simulink model "DIPCalt"  (R2015a)
settings: Solver=ode3  SolverMode=SingleTasking  StartTime=0.0  StopTime=5  FixedStep=1e-3  RelTol=1e-3
values from neighbouring files (symbols this model uses):
  deltas = ds/20    (= 45)    [DIPCinit.m]
  deltav = 1500    [DIPCinit.m]
  ds = 900    [DIPCinit.m]
  dv = 1500    [DIPCinit.m]
  g = [0;0;0]    [DIPCinit.m]
  j0 = 0.2    [DIPCinit.m]
  j1 = 0.5    [DIPCinit.m]
  j2 = 0.5    [DIPCinit.m]
  j3 = 0.5    [DIPCinit.m]
  j4 = 0.5    [DIPCinit.m]
  jiv = 0.5    [DIPCinit.m]
  jv = j0*1    (= 0.2)    [DIPCinit.m]
  kappas = ks/20    (= 9)    [DIPCinit.m]
  kappav = 700    [DIPCinit.m]
  ks = 180    [DIPCinit.m]
  kv = 700    [DIPCinit.m]
  m0 = 1.4    [DIPCinit.m]
  m1 = 10    [DIPCinit.m]
  m2 = 10    [DIPCinit.m]
  m3 = 10    [DIPCinit.m]
  m4 = 10    [DIPCinit.m]
  miv = 10    [DIPCinit.m]
  mv = m0*1    (= 1.4)    [DIPCinit.m]
  r = 0.4*[1 0 0 0 1 0 -1 0 0 0 -1 0]'    [DIPCinit.m]
libraries: aerolibutil x20, dspinverses x4, simulink x3, aerolibtransform2 x2
(part 1 of 2)
settings Model: CovSFcnEnable=off  Creator=Martin  LastModifiedBy=mangerer
settings OptimizationCC: BlockReduction=off  BooleanDataType=off  OptimizeBlockIOStorage=off  BufferReuse=off  GlobalBufferReuse=off  ExpressionFolding=off  LocalBlockOutputs=off
settings DebuggingCC: SaveWithParameterizedLinksMsg=none  UnderspecifiedInitializationDetection=Classic  MergeDetectMultiDrivingBlocksExec=none  SignalResolutionControl=TryResolveAllWithWarning
settings HardwareCC: TargetUnknown=on

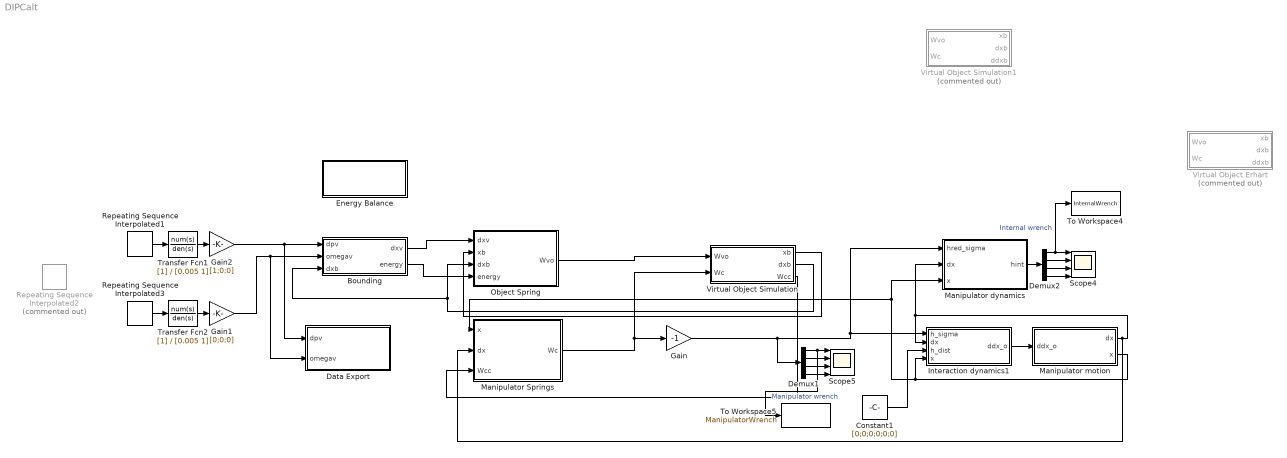
== system DIPCalt ==
  Bounding : Subsystem
  Constant1 : Constant  Value=[0;0;0;0;0;0]
  Data Export : Subsystem
  Demux1 : Demux
  Demux2 : Demux
  Energy Balance : Subsystem
  Gain : Gain  Gain=-1
  Gain1 : Gain  Gain=[0;0;0]
  Gain2 : Gain  Gain=[1;0;0]
  Interaction dynamics1 : Subsystem
  Manipulator Springs : Subsystem
  Manipulator dynamics : Subsystem
  Manipulator motion : Subsystem
  Object Spring : Subsystem
  Repeating Sequence Interpolated1 : simulink/Sources/Repeating Sequence Interpolated  OutValues="[0 0 0.2 0, 0 1 0, 0  -0.5 0, 0].'"  TimeValues=5/3*[0 0.1 0.25 0.4, 0.5 1.2 1.95, 2.15 2.45 2.85, 3].'  LookUpMeth=Interpolation-Use End Values  tsamp=0.001  OutMin=[]  OutMax=[]  OutDataTypeStr=double  OutputDataTypeScalingMode=double  OutDataType=fixdt(0,8)  OutScaling=2^-10
  Repeating Sequence Interpolated2 : simulink/Sources/Repeating Sequence Interpolated  Commented=on  OutValues=[0 0 2 2 -0.5 -0.5 0 0].'  TimeValues=[0 0.1 1 1.3 1.9 2.2 2.7 3].'  LookUpMeth=Interpolation-Use End Values  tsamp=0.001  OutMin=[]  OutMax=[]  OutDataTypeStr=double  OutputDataTypeScalingMode=double  OutDataType=fixdt(0,8)  OutScaling=2^-10
  Repeating Sequence Interpolated3 : simulink/Sources/Repeating Sequence Interpolated  OutValues="[0 0 0.2 0, 0 1 0, 0  -0.5 0, 0].'"  TimeValues=5/3*[0 0.1 0.25 0.4, 0.5 1.2 1.95, 2.15 2.45 2.85, 3].'  LookUpMeth=Interpolation-Use End Values  tsamp=0.001  OutMin=[]  OutMax=[]  OutDataTypeStr=double  OutputDataTypeScalingMode=double  OutDataType=fixdt(0,8)  OutScaling=2^-10
  Scope4 : Scope  NumInputPorts=4
      settings: ShowLegends=on  TimeRange=5  YMin=-2.25~-2.25~-1.5~-1.5  YMax=1.5~1.5~2.25~2.25  SaveName=ScopeData6
  Scope5 : Scope  NumInputPorts=4
      settings: ShowLegends=on  TimeRange=5  YMin=-12.5~-12.5~-20~-20  YMax=20~20~12.5~12.5  SaveName=ScopeData11
  To Workspace4 : ToWorkspace  VariableName=InternalWrench  SaveFormat=Timeseries  SampleTime=-1
  To Workspace5 : ToWorkspace  VariableName=ManipulatorWrench  SaveFormat=Timeseries  SampleTime=-1
  Transfer Fcn1 : TransferFcn  Denominator=[0.005 1]
  Transfer Fcn2 : TransferFcn  Denominator=[0.005 1]
  Virtual Object Erhart : Subsystem  Commented=on
  Virtual Object Simulation : Subsystem
  Virtual Object Simulation1 : Subsystem  Commented=on
  wires:
  Object Spring/1(Wvo) -> Virtual Object Simulation/1(Wvo)
  Virtual Object Simulation/1(xb) -> Object Spring/2(xb)
  Manipulator Springs/1(Wc) -> Virtual Object Simulation/2(Wc), Gain/1
  Interaction dynamics1/1(ddx_o) -> Manipulator motion/1(ddx_o)
  Constant1/1 -> Interaction dynamics1/3(h_dist)
  Manipulator motion/1(dx) -> Manipulator Springs/2(dx), Manipulator dynamics/2(dx), Interaction dynamics1/2(dx)
  Manipulator motion/2(x) -> Manipulator dynamics/3(x), Manipulator Springs/1(x), Interaction dynamics1/4(x)
  Virtual Object Simulation/2(dxb) -> Object Spring/3(dxb), Bounding/3(dxb)
  Manipulator dynamics/1(hint) -> Demux2/1
  Demux2/2 -> Scope4/2
  Demux2/4 -> Scope4/4
  Demux2/3 -> Scope4/3
  Demux2/1 -> To Workspace4/1, Scope4/1  "Internal wrench"
  Repeating Sequence Interpolated1/1 -> Transfer Fcn1/1
  Transfer Fcn1/1 -> Gain2/1
  Transfer Fcn2/1 -> Gain1/1
  Gain/1 -> Demux1/1, Manipulator dynamics/1(hred_sigma), Interaction dynamics1/1(h_sigma)
  Demux1/2 -> Scope5/2
  Demux1/4 -> Scope5/4
  Demux1/3 -> Scope5/3
  Demux1/1 -> To Workspace5/1, Scope5/1  "Manipulator wrench"
  Gain1/1 -> Data Export/2(omegav), Bounding/2(omegav)
  Gain2/1 -> Data Export/1(dpv), Bounding/1(dpv)
  Bounding/1(dxv) -> Object Spring/1(dxv)
  Bounding/2(energy) -> Object Spring/4(energy)
  Repeating Sequence Interpolated3/1 -> Transfer Fcn2/1
  Virtual Object Simulation/3(Wcc) -> Manipulator Springs/3(Wcc)

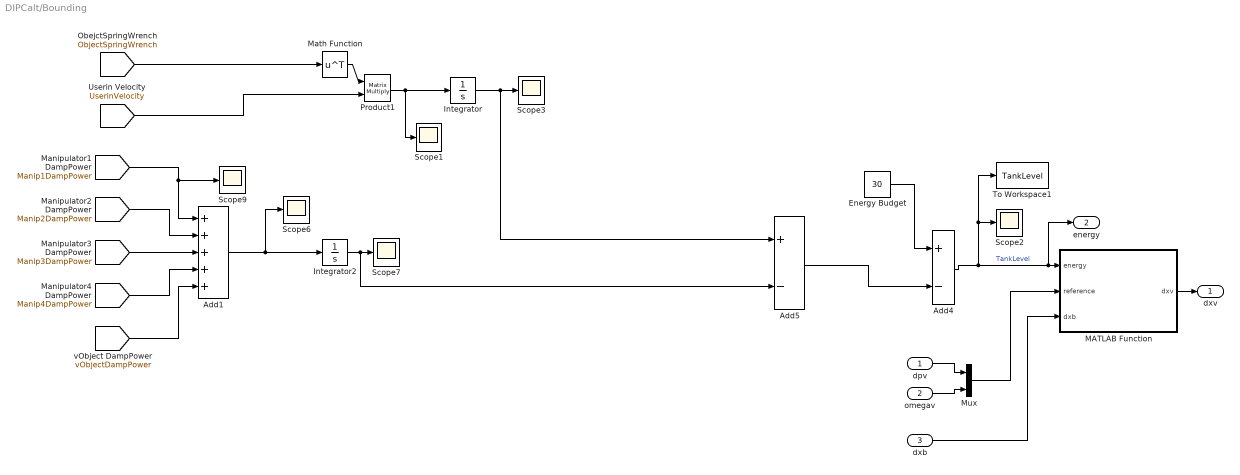
== system DIPCalt/Bounding ==
  dpv : Inport
  omegav : Inport  Port=2
  dxb : Inport  Port=3
  Add1 : Sum  Inputs=+++++
  Add4 : Sum  Inputs=+-
  Add5 : Sum  Inputs=+-
  Energy Budget : Constant  Value=30
  Integrator : Integrator
  Integrator2 : Integrator
  MATLAB Function : MATLAB Function  TreatAsAtomicUnit=on
  Math Function : Math  Operator=transpose  SaturateOnIntegerOverflow=on
  Mux : Mux  Inputs=2
  Product1 : Product  Multiplication=Matrix(*)
  Scope{1..3,6..7,9} (6 alike) : Scope
      Scope1 settings: YMin=0  YMax=60  SaveName=ScopeData5
      Scope2 settings: TimeRange=4.999  YMin=19.5  YMax=30
      Scope3 settings: YMin=0  YMax=15  SaveName=ScopeData14
      Scope6 settings: YMin=-0.3  YMax=0.05  SaveName=ScopeData40
      Scope7 settings: YMin=675  YMax=1000  SaveName=ScopeData41
      Scope9 settings: YMin=0  YMax=3e-05  SaveName=ScopeData46
  To Workspace1 : ToWorkspace  VariableName=TankLevel  SaveFormat=Timeseries  SampleTime=-1
  dxv : Outport
  energy : Outport  Port=2
  wires:
  Energy Budget/1 -> Add4/1
  Add4/1 -> energy/1, MATLAB Function/1(energy), To Workspace1/1, Scope2/1  "TankLevel"
  dpv/1 -> Mux/1
  omegav/1 -> Mux/2
  Mux/1 -> MATLAB Function/2(reference)
  dxb/1 -> MATLAB Function/3(dxb)
  MATLAB Function/1(dxv) -> dxv/1
  Product1/1 -> Integrator/1, Scope1/1
  [UserinVelocity] -> Product1/2
  Integrator/1 -> Add5/1, Scope3/1
  [Manip1DampPower] -> Scope9/1, Add1/1
  [Manip2DampPower] -> Add1/2
  [Manip3DampPower] -> Add1/3
  [Manip4DampPower] -> Add1/4
  [vObjectDampPower] -> Add1/5
  Add1/1 -> Integrator2/1, Scope6/1
  Integrator2/1 -> Add5/2, Scope7/1
  Math Function/1 -> Product1/1
  [ObjectSpringWrench] -> Math Function/1
  Add5/1 -> Add4/2

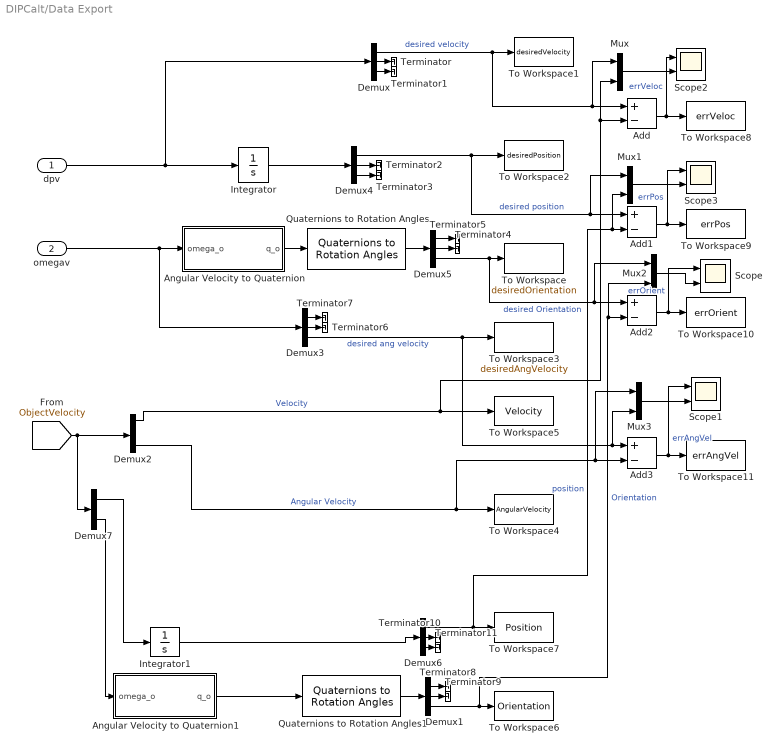
== system DIPCalt/Data Export ==
  dpv : Inport
  omegav : Inport  Port=2
  Add{,1..3} (4 alike) : Sum  Inputs=+-
  Angular Velocity to Quaternion : Subsystem
  Angular Velocity to Quaternion1 : Subsystem
  Demux{,1,3..6} (6 alike) : Demux  Outputs=3
  Demux2 : Demux  Outputs=6
  Demux7 : Demux  Outputs=2
  Integrator : Integrator
  Integrator1 : Integrator  InitialCondition=[0 0 0]'
  Mux{,1..3} (4 alike) : Mux  Inputs=2
  Quaternions to Rotation Angles : aerolibtransform2/Quaternions to Rotation Angles  rotationOrder=XYZ
  Quaternions to Rotation Angles1 : aerolibtransform2/Quaternions to Rotation Angles  rotationOrder=XYZ
  Scope{,1..3} (4 alike) : Scope  NumInputPorts=2
      Scope settings: YMin=-0.0005~-5  YMax=0.0025~5  SaveName=ScopeData13
      Scope1 settings: YMin=-0.06~-0.025  YMax=0.08~0.225  SaveName=ScopeData37
      Scope2 settings: TimeRange=4.999  YMin=-0.3~-0.5  YMax=0.2~1  SaveName=ScopeData19
      Scope3 settings: YMin=-0.0005~-5  YMax=0.0025~5  SaveName=ScopeData39
  Terminator{,1..11} (12 alike) : Terminator
  To Workspace : ToWorkspace  VariableName=desiredOrientation  SaveFormat=Timeseries  SampleTime=-1
  To Workspace1 : ToWorkspace  VariableName=desiredVelocity  SaveFormat=Timeseries  SampleTime=-1
  To Workspace10 : ToWorkspace  VariableName=errOrient  SaveFormat=Timeseries  SampleTime=-1
  To Workspace11 : ToWorkspace  VariableName=errAngVel  SaveFormat=Timeseries  SampleTime=-1
  To Workspace2 : ToWorkspace  VariableName=desiredPosition  SaveFormat=Timeseries  SampleTime=-1
  To Workspace3 : ToWorkspace  VariableName=desiredAngVelocity  SaveFormat=Timeseries  SampleTime=-1
  To Workspace4 : ToWorkspace  VariableName=AngularVelocity  SaveFormat=Timeseries  SampleTime=-1
  To Workspace5 : ToWorkspace  VariableName=Velocity  SaveFormat=Timeseries  SampleTime=-1
  To Workspace6 : ToWorkspace  VariableName=Orientation  SaveFormat=Timeseries  SampleTime=-1
  To Workspace7 : ToWorkspace  VariableName=Position  SaveFormat=Timeseries  SampleTime=-1
  To Workspace8 : ToWorkspace  VariableName=errVeloc  SaveFormat=Timeseries  SampleTime=-1
  To Workspace9 : ToWorkspace  VariableName=errPos  SaveFormat=Timeseries  SampleTime=-1
  wires:
  Demux4/1 -> Mux1/1, Add1/1, To Workspace2/1  "desired position"
  Demux/1 -> Mux/1, Add/1, To Workspace1/1  "desired velocity"
  Integrator/1 -> Demux4/1
  dpv/1 -> Demux/1, Integrator/1
  Demux/2 -> Terminator/1
  Demux/3 -> Terminator1/1
  Demux4/2 -> Terminator2/1
  Demux4/3 -> Terminator3/1
  Quaternions to Rotation Angles/1 -> Demux5/1
  Demux5/3 -> Mux2/1, Add2/1, To Workspace/1  "desired Orientation"
  Demux3/3 -> Mux3/2, Add3/1, To Workspace3/1  "desired ang velocity"
  Angular Velocity to Quaternion/1(q_o) -> Quaternions to Rotation Angles/1
  omegav/1 -> Demux3/1, Angular Velocity to Quaternion/1(omega_o)
  Demux5/2 -> Terminator4/1
  Demux5/1 -> Terminator5/1
  Demux3/2 -> Terminator6/1
  Demux3/1 -> Terminator7/1
  Demux2/1 -> Mux/2, Add/2, To Workspace5/1  "Velocity"
  Demux2/6 -> Mux3/1, Add3/2, To Workspace4/1  "Angular Velocity"
  [ObjectVelocity] -> Demux7/1, Demux2/1
  Quaternions to Rotation Angles1/1 -> Demux1/1
  Demux1/3 -> Mux2/2, Add2/2, To Workspace6/1  "Orientation"
  Demux1/2 -> Terminator9/1
  Demux1/1 -> Terminator8/1
  Demux6/1 -> Mux1/2, Add1/2, To Workspace7/1  "position"
  Demux6/2 -> Terminator10/1
  Demux6/3 -> Terminator11/1
  Demux7/1 -> Integrator1/1
  Integrator1/1 -> Demux6/1
  Demux7/2 -> Angular Velocity to Quaternion1/1(omega_o)
  Angular Velocity to Quaternion1/1(q_o) -> Quaternions to Rotation Angles1/1
  Add/1 -> Scope2/1, To Workspace8/1  "errVeloc"
  Add1/1 -> Scope3/1, To Workspace9/1  "errPos"
  Add2/1 -> Scope/1, To Workspace10/1  "errOrient"
  Add3/1 -> Scope1/1, To Workspace11/1  "errAngVel"
  Mux/1 -> Scope2/2
  Mux1/1 -> Scope3/2
  Mux2/1 -> Scope/2
  Mux3/1 -> Scope1/2

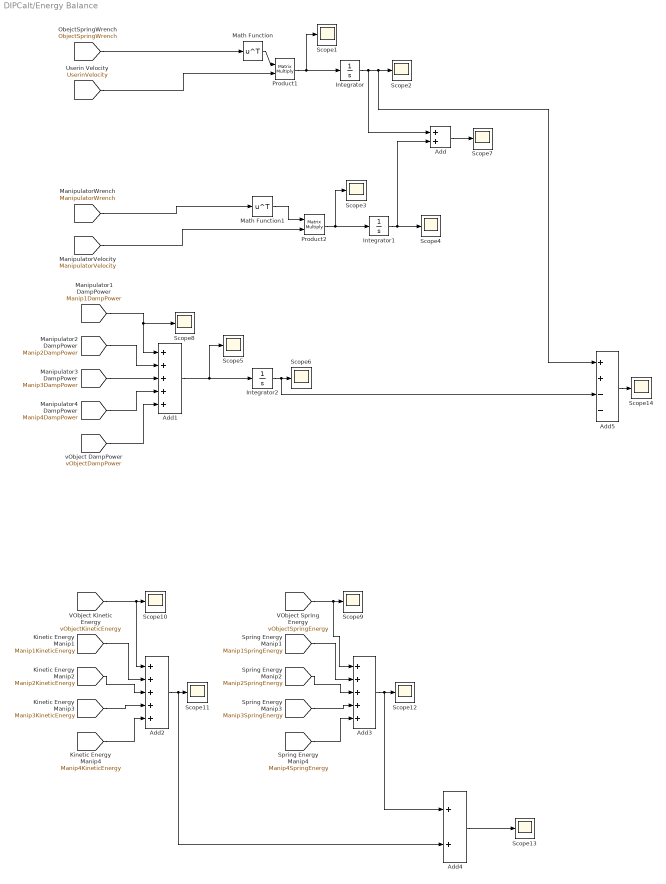
== system DIPCalt/Energy Balance ==
  Add : Sum
  Add1 : Sum  Inputs=+++++
  Add2 : Sum  Inputs=+++++
  Add3 : Sum  Inputs=+++++
  Add4 : Sum
  Add5 : Sum  Inputs=++--
  Integrator : Integrator
  Integrator1 : Integrator
  Integrator2 : Integrator
  Math Function : Math  Operator=transpose  SaturateOnIntegerOverflow=on
  Math Function1 : Math  Operator=transpose  SaturateOnIntegerOverflow=on
  Product1 : Product  Multiplication=Matrix(*)
  Product2 : Product  Multiplication=Matrix(*)
  Scope{1..14} (14 alike) : Scope
      Scope1 settings: YMin=0  YMax=60  SaveName=ScopeData24
      Scope10 settings: YMin=0  YMax=0.08  SaveName=ScopeData29
      Scope11 settings: YMin=0  YMax=12  SaveName=ScopeData30
      Scope12 settings: YMin=0  YMax=0.00021  SaveName=ScopeData31
      Scope13 settings: YMin=0  YMax=50  SaveName=ScopeData32
      Scope14 settings: YMin=0  YMax=42.5  SaveName=ScopeData33
      Scope2 settings: YMin=0  YMax=15  SaveName=ScopeData18
      Scope3 settings: YMin=-60  YMax=10  SaveName=ScopeData20
      Scope4 settings: YMin=1  YMax=4.5  SaveName=ScopeData21
      Scope5 settings: YMin=-0.3  YMax=0.05  SaveName=ScopeData22
      Scope6 settings: YMin=675  YMax=1000  SaveName=ScopeData25
      Scope7 settings: YMin=0  YMax=25  SaveName=ScopeData26
      Scope8 settings: YMin=0  YMax=3e-05  SaveName=ScopeData27
      Scope9 settings: YMin=-4.16334e-17  YMax=0.575  SaveName=ScopeData28
  wires:
  Product1/1 -> Integrator/1, Scope1/1
  [UserinVelocity] -> Product1/2
  Integrator/1 -> Add/1, Add5/1, Scope2/1
  Product2/1 -> Integrator1/1, Scope3/1
  Math Function1/1 -> Product2/1
  [ManipulatorVelocity] -> Product2/2
  Integrator1/1 -> Add/2, Scope4/1
  Add/1 -> Scope7/1
  [Manip1DampPower] -> Scope8/1, Add1/1
  [Manip2DampPower] -> Add1/2
  [Manip3DampPower] -> Add1/3
  [Manip4DampPower] -> Add1/4
  [vObjectDampPower] -> Add1/5
  Add1/1 -> Integrator2/1, Scope5/1
  [vObjectSpringEnergy] -> Add3/1, Scope9/1
  [vObjectKineticEnergy] -> Add2/1, Scope10/1
  Add2/1 -> Add4/2, Scope11/1
  Add3/1 -> Add4/1, Scope12/1
  Add4/1 -> Scope13/1
  Integrator2/1 -> Add5/3, Scope6/1
  Add5/1 -> Scope14/1
  Math Function/1 -> Product1/1
  [ObjectSpringWrench] -> Math Function/1
  [ManipulatorWrench] -> Math Function1/1
  [Manip4KineticEnergy] -> Add2/5
  [Manip4SpringEnergy] -> Add3/5
  [Manip3SpringEnergy] -> Add3/4
  [Manip2SpringEnergy] -> Add3/3
  [Manip1SpringEnergy] -> Add3/2
  [Manip3KineticEnergy] -> Add2/4
  [Manip2KineticEnergy] -> Add2/3
  [Manip1KineticEnergy] -> Add2/2

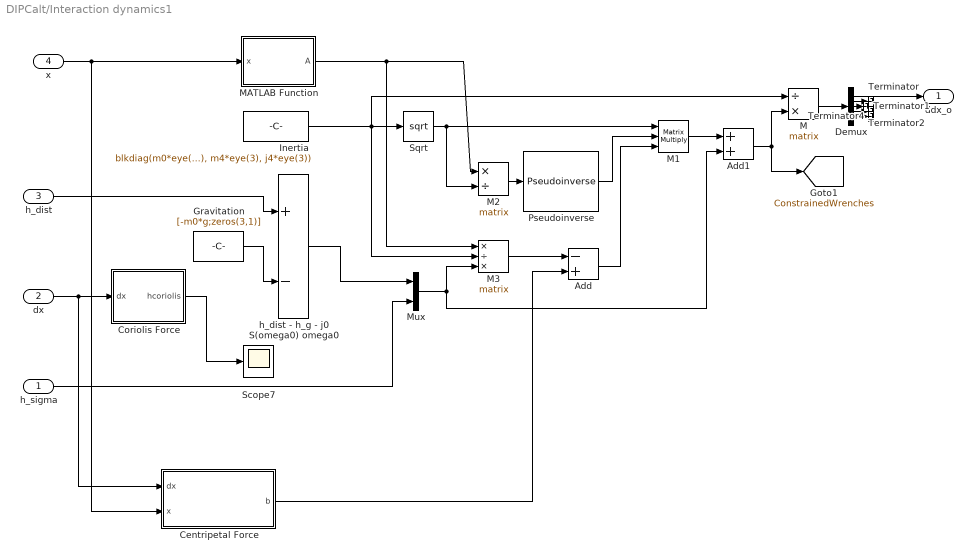
== system DIPCalt/Interaction dynamics1 ==
  h_sigma : Inport
  dx : Inport  Port=2
  h_dist : Inport  Port=3
  x : Inport  Port=4
  Add : Sum  Inputs=-+
  Add1 : Sum
  Centripetal Force : MATLAB Function  TreatAsAtomicUnit=on
  Coriolis Force : MATLAB Function  TreatAsAtomicUnit=on
  Demux : Demux  Outputs=5
  Gravitation : Constant  Value=[-m0*g;zeros(3,1)]
  Inertia : Constant  Value=blkdiag(m0*eye(3),j0*eye(3),m1*eye(3), j1*eye(3), m2*eye(3), j2*eye(3),m3*eye(3), j3*eye(3), m4*eye(3), j4*eye(3))
  M : Product  Inputs=/*  Multiplication=Matrix(*)
  M1 : Product  Inputs=***  Multiplication=Matrix(*)
  M2 : Product  Inputs=*/  Multiplication=Matrix(*)
  M3 : Product  Inputs=*/*  Multiplication=Matrix(*)
  MATLAB Function : MATLAB Function  TreatAsAtomicUnit=on
  Mux : Mux  Inputs=2
  Pseudoinverse : dspinverses/Pseudoinverse  wanterr=off
  Scope7 : Scope
      settings: YMin=-0.1  YMax=1.2  SaveName=ScopeData3
  Sqrt : Sqrt  SaturateOnIntegerOverflow=on
  Terminator{,1..2,4} (4 alike) : Terminator
  "h_dist - h_g - j0 S(omega0) omega0 " : Sum  Inputs=+-
  ddx_o : Outport
  tag scope: ConstrainedWrenches=global
  wires:
  h_dist/1 -> "h_dist - h_g - j0 S(omega0) omega0 "/1
  Gravitation/1 -> "h_dist - h_g - j0 S(omega0) omega0 "/2
  dx/1 -> Centripetal Force/1(dx), Coriolis Force/1(dx)
  Coriolis Force/1(hcoriolis) -> Scope7/1
  x/1 -> MATLAB Function/1(x), Centripetal Force/2(x)
  Inertia/1 -> M/1, M3/2, Sqrt/1
  Sqrt/1 -> M2/2, M1/1
  MATLAB Function/1(A) -> M3/1, M2/1
  M2/1 -> Pseudoinverse/1
  Pseudoinverse/1 -> M1/2
  Add/1 -> M1/3
  Centripetal Force/1(b) -> Add/2
  M3/1 -> Add/1
  Mux/1 -> Add1/2, M3/3
  "h_dist - h_g - j0 S(omega0) omega0 "/1 -> Mux/1
  h_sigma/1 -> Mux/2
  M/1 -> Demux/1
  Demux/1 -> ddx_o/1
  M1/1 -> Add1/1
  Add1/1 -> M/2, [ConstrainedWrenches]
  Demux/2 -> Terminator/1
  Demux/3 -> Terminator1/1
  Demux/4 -> Terminator2/1
  Demux/5 -> Terminator4/1

== system DIPCalt/Manipulator Springs ==
  x : Inport
  dx : Inport  Port=2
  Wcc : Inport  Port=3
  Demux1 : Demux
  Demux2 : Demux
  Demux5 : Demux
  Mux : Mux
  Spring 1 : Subsystem
  Spring 2 : Subsystem
  Spring 3 : Subsystem
  Spring 4 : Subsystem
  Wc : Outport
  tag scope: ManipulatorWrench=global
  wires:
  Spring 1/1(Wc1) -> Mux/1
  Spring 2/1(Wc2) -> Mux/2
  Mux/1 -> Wc/1, [ManipulatorWrench]
  x/1 -> Demux1/1
  Spring 3/1(Wc3) -> Mux/3
  Spring 4/1(Wc4) -> Mux/4
  dx/1 -> Demux2/1
  Demux1/1 -> Spring 1/1(x1)
  Demux1/2 -> Spring 2/1(x2)
  Demux1/3 -> Spring 3/1(x3)
  Demux1/4 -> Spring 4/1(x4)
  Demux2/1 -> Spring 1/2(dx1)
  Demux2/2 -> Spring 2/2(dx2)
  Demux2/3 -> Spring 3/2(dx3)
  Demux2/4 -> Spring 4/2(dx4)
  Wcc/1 -> Demux5/1
  Demux5/1 -> Spring 1/3(Wcc1)
  Demux5/2 -> Spring 2/3(Wcc2)
  Demux5/3 -> Spring 3/3(Wcc3)
  Demux5/4 -> Spring 4/3(Wcc4)

== system DIPCalt/Manipulator dynamics ==
  hred_sigma : Inport
  dx : Inport  Port=2
  x : Inport  Port=3
  A_ * M * A_' : Product  Commented=on  Inputs=*/*  Multiplication=Matrix(*)
  A_'(A_ *M *A_')^-1(b_ - A_/M*hred) : Product  Commented=on  Inputs=*/*  Multiplication=Matrix(*)
  A_/M*hred : Product  Inputs=*/*  Multiplication=Matrix(*)
  Centripal Force : MATLAB Function  TreatAsAtomicUnit=on
  Inertia : Constant  Value=blkdiag(m1*eye(3), j1*eye(3), m2*eye(3), j2*eye(3), m3*eye(3), j3*eye(3), m4*eye(3), j4*eye(3))
  Mult : Product  Inputs=***  Multiplication=Matrix(*)
  Mult1 : Product  Inputs=*/  Multiplication=Matrix(*)
  Pseudoinverse : dspinverses/Pseudoinverse  wanterr=off
  Reduced Constraint Matrix : MATLAB Function  TreatAsAtomicUnit=on
  Sqrt : Sqrt  SaturateOnIntegerOverflow=on
  World to Object Frame : MATLAB Function  TreatAsAtomicUnit=on
  b_ - A_/M*hred : Sum  Inputs=-+
  hint : Outport
  wires:
  Reduced Constraint Matrix/1(Ared) -> A_/M*hred/1, Mult1/1
  Inertia/1 -> Sqrt/1, A_/M*hred/2
  dx/1 -> Centripal Force/2(dx)
  A_/M*hred/1 -> b_ - A_/M*hred/1
  hred_sigma/1 -> A_/M*hred/3
  World to Object Frame/1(h_int) -> hint/1
  x/1 -> Centripal Force/1(x), Reduced Constraint Matrix/1(x), World to Object Frame/2(x)
  Centripal Force/1(bred) -> b_ - A_/M*hred/2
  Mult/1 -> World to Object Frame/1(hw)
  b_ - A_/M*hred/1 -> Mult/3
  Sqrt/1 -> Mult1/2, Mult/1
  Mult1/1 -> Pseudoinverse/1
  Pseudoinverse/1 -> Mult/2

== system DIPCalt/Manipulator motion ==
  ddx_o : Inport
  Angular Velocity to Quaternion : Subsystem
  Demux : Demux  Outputs=2
  G' dx_o : Product  Multiplication=Matrix(*)
  Grasp Matrix : MATLAB Function  TreatAsAtomicUnit=on
  Integrator : Integrator  InitialCondition=zeros(6,1)
  Integrator1 : Integrator  InitialCondition=[0 0 0]'
  Manipualtor pose in world frame : MATLAB Function  TreatAsAtomicUnit=on
  Scope3 : Scope
      settings: SaveName=ScopeData7
  Scope4 : Scope
      settings: YMin=-0.45  YMax=0.05  SaveName=ScopeData16
  Transpose : Math  Operator=transpose  SaturateOnIntegerOverflow=on
  dx : Outport
  x : Outport  Port=2
  tag scope: ManipulatorPose=global, ManipulatorVelocity=global, ObjectVelocity=global
  wires:
  ddx_o/1 -> Scope3/1, Integrator/1
  Integrator/1 -> Scope4/1, [ObjectVelocity], G' dx_o/2, Demux/1
  Grasp Matrix/1(G) -> Transpose/1
  Transpose/1 -> G' dx_o/1
  G' dx_o/1 -> [ManipulatorVelocity], dx/1
  Demux/2 -> Angular Velocity to Quaternion/1(omega_o)
  Demux/1 -> Integrator1/1
  Integrator1/1 -> Manipualtor pose in world frame/1(p_o)
  Manipualtor pose in world frame/1(x) -> [ManipulatorPose], Grasp Matrix/1(x), x/1
  Angular Velocity to Quaternion/1(q_o) -> Manipualtor pose in world frame/2(q_o)

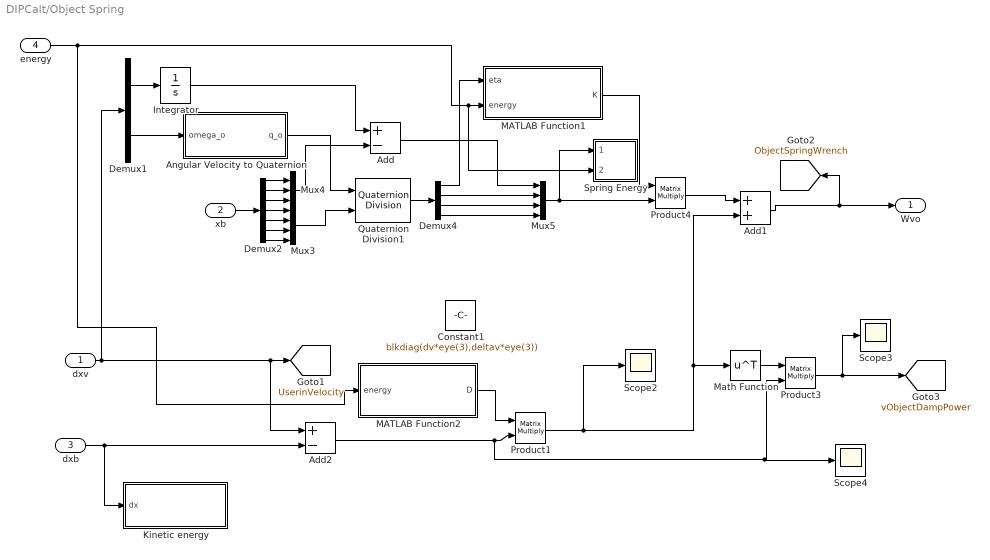
== system DIPCalt/Object Spring ==
  dxv : Inport
  xb : Inport  Port=2
  dxb : Inport  Port=3
  energy : Inport  Port=4
  Add : Sum  Inputs=+-
  Add1 : Sum
  Add2 : Sum  Inputs=+-
  Angular Velocity to Quaternion : Subsystem
  Constant1 : Constant  Value=blkdiag(dv*eye(3),deltav*eye(3))
  Demux1 : Demux  Outputs=2
  Demux2 : Demux  Outputs=7
  Demux4 : Demux
  Integrator : Integrator
  Kinetic energy : Subsystem
  MATLAB Function1 : MATLAB Function  TreatAsAtomicUnit=on
  MATLAB Function2 : MATLAB Function  TreatAsAtomicUnit=on
  Math Function : Math  Operator=transpose  SaturateOnIntegerOverflow=on
  Mux3 : Mux
  Mux4 : Mux  Inputs=3
  Mux5 : Mux
  Product1 : Product  Multiplication=Matrix(*)
  Product3 : Product  Multiplication=Matrix(*)
  Product4 : Product  Multiplication=Matrix(*)
  Quaternion Division1 : aerolibutil/Quaternion Division
  Scope2 : Scope
      settings: YMin=-1500  YMax=6500  SaveName=ScopeData4
  Scope3 : Scope
      settings: YMin=0  YMax=8500  SaveName=ScopeData2
  Scope4 : Scope
      settings: YMin=-3.5  YMax=3  SaveName=ScopeData35
  Spring Energy : Subsystem
  Wvo : Outport
  tag scope: ObjectSpringWrench=global, UserinVelocity=global, vObjectDampPower=global
  wires:
  Add1/1 -> [ObjectSpringWrench], Wvo/1
  Product4/1 -> Add1/1
  Product1/1 -> Scope2/1, Math Function/1, Add1/2
  MATLAB Function1/1(K) -> Product4/1
  Demux4/1 -> MATLAB Function1/1(eta)
  Add/1 -> Mux5/1
  Demux4/2 -> Mux5/2
  Demux4/3 -> Mux5/3
  Demux4/4 -> Mux5/4
  Quaternion Division1/1 -> Demux4/1
  xb/1 -> Demux2/1
  Demux2/4 -> Mux3/1
  Demux2/5 -> Mux3/2
  Demux2/6 -> Mux3/3
  Demux2/7 -> Mux3/4
  Demux2/1 -> Mux4/1
  Demux2/2 -> Mux4/2
  Demux2/3 -> Mux4/3
  Mux4/1 -> Add/2
  Mux3/1 -> Quaternion Division1/2
  Add2/1 -> Scope4/1, Product3/2, Product1/2
  dxv/1 -> Demux1/1, [UserinVelocity], Add2/1
  dxb/1 -> Kinetic energy/1(dx), Add2/2
  Product3/1 -> Scope3/1, [vObjectDampPower]
  Math Function/1 -> Product3/1
  Mux5/1 -> Spring Energy/1(deltax), Product4/2
  Demux1/1 -> Integrator/1
  Integrator/1 -> Add/1
  Demux1/2 -> Angular Velocity to Quaternion/1(omega_o)
  Angular Velocity to Quaternion/1(q_o) -> Quaternion Division1/1
  energy/1 -> Spring Energy/2(energy), MATLAB Function1/2(energy), MATLAB Function2/1(energy)
  MATLAB Function2/1(D) -> Product1/1

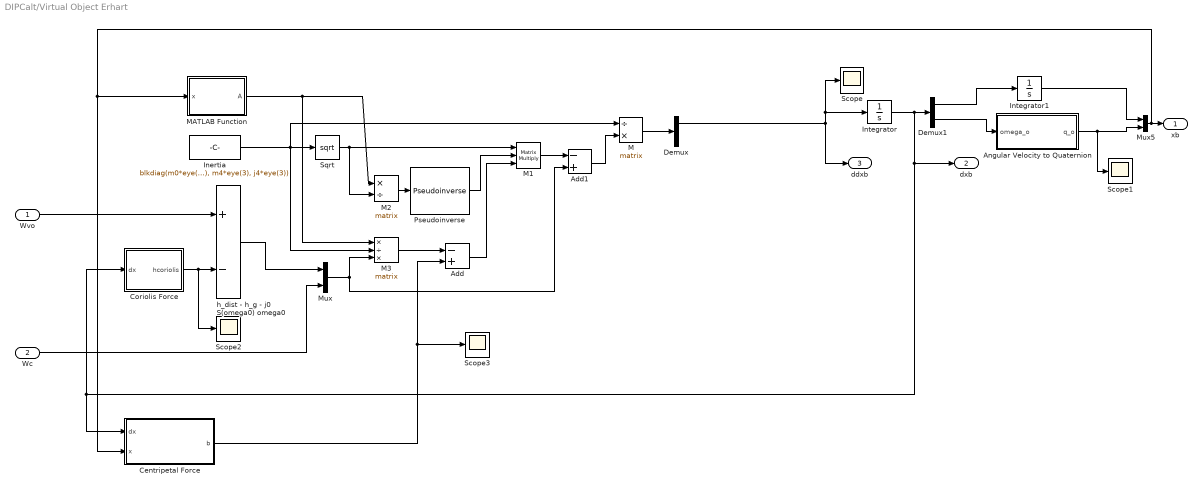
== system DIPCalt/Virtual Object Erhart ==
  Wvo : Inport
  Wc : Inport  Port=2
  Add : Sum  Inputs=-+
  Add1 : Sum  Inputs=-+
  Angular Velocity to Quaternion : Subsystem
  Centripetal Force : MATLAB Function  TreatAsAtomicUnit=on
  Coriolis Force : MATLAB Function  TreatAsAtomicUnit=on
  Demux : Demux  Outputs=5
  Demux1 : Demux  Outputs=2
  Inertia : Constant  Value=blkdiag(m0*eye(3),j0*eye(3),m1*eye(3), j1*eye(3), m2*eye(3), j2*eye(3),m3*eye(3), j3*eye(3), m4*eye(3), j4*eye(3))
  Integrator : Integrator  InitialCondition=zeros(6,1)
  Integrator1 : Integrator  InitialCondition=[0 0 0]'
  M : Product  Inputs=/*  Multiplication=Matrix(*)
  M1 : Product  Inputs=***  Multiplication=Matrix(*)
  M2 : Product  Inputs=*/  Multiplication=Matrix(*)
  M3 : Product  Inputs=*/*  Multiplication=Matrix(*)
  MATLAB Function : MATLAB Function  TreatAsAtomicUnit=on
  Mux : Mux  Inputs=2
  Mux5 : Mux  Inputs=2
  Pseudoinverse : dspinverses/Pseudoinverse  wanterr=off
  Scope{,1..3} (4 alike) : Scope
      Scope1 settings: SaveName=ScopeData8
      Scope2 settings: SaveName=ScopeData15
      Scope3 settings: YMin=-1  YMax=1  SaveName=ScopeData17
  Sqrt : Sqrt  SaturateOnIntegerOverflow=on
  "h_dist - h_g - j0 S(omega0) omega0 " : Sum  Inputs=+-
  xb : Outport
  dxb : Outport  Port=2
  ddxb : Outport  Port=3
  wires:
  Demux/1 -> Scope/1, Integrator/1, ddxb/1
  Integrator/1 -> Demux1/1, Coriolis Force/1(dx), Centripetal Force/1(dx), dxb/1
  Demux1/2 -> Angular Velocity to Quaternion/1(omega_o)
  Demux1/1 -> Integrator1/1
  Integrator1/1 -> Mux5/1
  Angular Velocity to Quaternion/1(q_o) -> Scope1/1, Mux5/2
  Wvo/1 -> "h_dist - h_g - j0 S(omega0) omega0 "/1
  Coriolis Force/1(hcoriolis) -> Scope2/1, "h_dist - h_g - j0 S(omega0) omega0 "/2
  Mux5/1 -> MATLAB Function/1(x), Centripetal Force/2(x), xb/1
  Inertia/1 -> M/1, M3/2, Sqrt/1
  Sqrt/1 -> M2/2, M1/1
  MATLAB Function/1(A) -> M3/1, M2/1
  M2/1 -> Pseudoinverse/1
  Pseudoinverse/1 -> M1/2
  Add/1 -> M1/3
  Centripetal Force/1(b) -> Scope3/1, Add/2
  M3/1 -> Add/1
  Mux/1 -> Add1/2, M3/3
  "h_dist - h_g - j0 S(omega0) omega0 "/1 -> Mux/1
  Wc/1 -> Mux/2
  M1/1 -> Add1/1
  Add1/1 -> M/2
  M/1 -> Demux/1

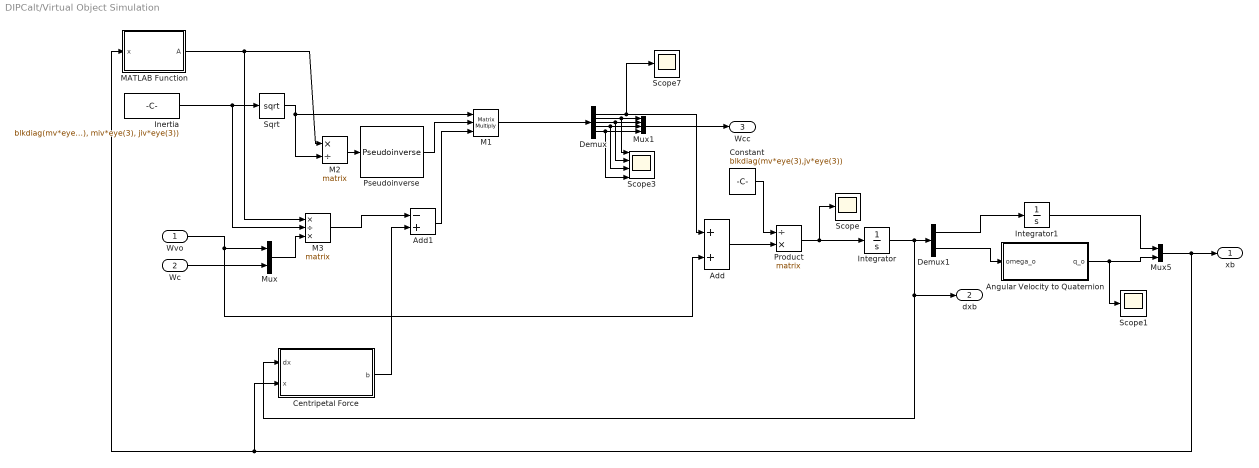
== system DIPCalt/Virtual Object Simulation ==
  Wvo : Inport
  Wc : Inport  Port=2
  Add : Sum
  Add1 : Sum  Inputs=-+
  Angular Velocity to Quaternion : Subsystem
  Centripetal Force : MATLAB Function  TreatAsAtomicUnit=on
  Constant : Constant  Value=blkdiag(mv*eye(3),jv*eye(3))
  Demux : Demux  Outputs=5
  Demux1 : Demux  Outputs=2
  Inertia : Constant  Value=blkdiag(mv*eye(3),jv*eye(3),miv*eye(3), jiv*eye(3), miv*eye(3), jiv*eye(3),miv*eye(3), jiv*eye(3), miv*eye(3), jiv*eye(3))
  Integrator : Integrator  InitialCondition=zeros(6,1)
  Integrator1 : Integrator  InitialCondition=[0 0 0]'
  M1 : Product  Inputs=***  Multiplication=Matrix(*)
  M2 : Product  Inputs=*/  Multiplication=Matrix(*)
  M3 : Product  Inputs=*/*  Multiplication=Matrix(*)
  MATLAB Function : MATLAB Function  TreatAsAtomicUnit=on
  Mux : Mux  Inputs=2
  Mux1 : Mux
  Mux5 : Mux  Inputs=2
  Product : Product  Inputs=/*  Multiplication=Matrix(*)
  Pseudoinverse : dspinverses/Pseudoinverse  wanterr=off
  Scope : Scope
      settings: YMin=-3  YMax=4
  Scope1 : Scope
      settings: SaveName=ScopeData8
  Scope3 : Scope  NumInputPorts=4
      settings: YMin=-400~-400~-400~-400  YMax=700~700~700~700  SaveName=ScopeData36
  Scope7 : Scope
      settings: YMin=-0.1  YMax=1.2  SaveName=ScopeData42
  Sqrt : Sqrt  SaturateOnIntegerOverflow=on
  xb : Outport
  dxb : Outport  Port=2
  Wcc : Outport  Port=3
  wires:
  Add/1 -> Product/2
  Constant/1 -> Product/1
  Product/1 -> Scope/1, Integrator/1
  Integrator/1 -> Demux1/1, Centripetal Force/1(dx), dxb/1
  Demux1/2 -> Angular Velocity to Quaternion/1(omega_o)
  Demux1/1 -> Integrator1/1
  Integrator1/1 -> Mux5/1
  Angular Velocity to Quaternion/1(q_o) -> Scope1/1, Mux5/2
  Mux5/1 -> Centripetal Force/2(x), MATLAB Function/1(x), xb/1
  Inertia/1 -> M3/2, Sqrt/1
  Sqrt/1 -> M2/2, M1/1
  MATLAB Function/1(A) -> M3/1, M2/1
  M2/1 -> Pseudoinverse/1
  Pseudoinverse/1 -> M1/2
  Add1/1 -> M1/3
  Mux/1 -> M3/3
  Demux/1 -> Scope7/1, Add/1
  Demux/5 -> Scope3/4, Mux1/4
  Demux/4 -> Scope3/3, Mux1/3
  Demux/3 -> Scope3/2, Mux1/2
  Demux/2 -> Scope3/1, Mux1/1
  Mux1/1 -> Wcc/1
  M1/1 -> Demux/1
  M3/1 -> Add1/1
  Centripetal Force/1(b) -> Add1/2
  Wvo/1 -> Add/2, Mux/1
  Wc/1 -> Mux/2

== system DIPCalt/Virtual Object Simulation1 ==
  Wvo : Inport
  Wc : Inport  Port=2
  Add : Sum  Inputs=+++
  Angular Velocity to Quaternion : Subsystem
  Constant : Constant  Value=blkdiag(mv*eye(3),jv*eye(3))
  Coriolis Force : MATLAB Function  TreatAsAtomicUnit=on
  Demux1 : Demux  Outputs=2
  Grasp Matrix : MATLAB Function  TreatAsAtomicUnit=on
  Integrator : Integrator  InitialCondition=zeros(6,1)
  Integrator1 : Integrator  InitialCondition=[0 0 0]'
  Mux5 : Mux  Inputs=2
  Product : Product  Inputs=/*  Multiplication=Matrix(*)
  Product1 : Product  Inputs=**  Multiplication=Matrix(*)
  Scope : Scope
  Scope1 : Scope
      settings: SaveName=ScopeData8
  Scope2 : Scope
      settings: YMin=-0.008  YMax=0.008  SaveName=ScopeData10
  xb : Outport
  dxb : Outport  Port=2
  ddxb : Outport  Port=3
  wires:
  Add/1 -> Product/2
  Constant/1 -> Product/1
  Product/1 -> ddxb/1, Scope/1, Integrator/1
  Integrator/1 -> Demux1/1, Coriolis Force/1(dx), dxb/1
  Demux1/2 -> Angular Velocity to Quaternion/1(omega_o)
  Demux1/1 -> Integrator1/1
  Integrator1/1 -> Mux5/1
  Angular Velocity to Quaternion/1(q_o) -> Scope1/1, Mux5/2
  Mux5/1 -> Grasp Matrix/1(x), xb/1
  Wvo/1 -> Add/1
  Product1/1 -> Add/2
  Grasp Matrix/1(G) -> Product1/1
  Wc/1 -> Product1/2
  Coriolis Force/1(hcoriolis) -> Scope2/1, Add/3

== system DIPCalt/Data Export/Angular Velocity to Quaternion ==
  omega_o : Inport
  Constant : Constant  Value=0
  Gain : Gain  Gain=0.5
  Integrator : Integrator  InitialCondition=[1; 0; 0; 0]
  Mux : Mux  Inputs=2
  Quaternion Multiplication : aerolibutil/Quaternion Multiplication
  Scope : Scope
      settings: ShowLegends=on  SaveName=ScopeData9
  q_o : Outport
  wires:
  omega_o/1 -> Gain/1
  Gain/1 -> Mux/2
  Constant/1 -> Mux/1
  Quaternion Multiplication/1 -> Integrator/1
  Integrator/1 -> Quaternion Multiplication/2, q_o/1, Scope/1
  Mux/1 -> Quaternion Multiplication/1

== system DIPCalt/Data Export/Angular Velocity to Quaternion1 ==
  omega_o : Inport
  Constant : Constant  Value=0
  Gain : Gain  Gain=0.5
  Integrator : Integrator  InitialCondition=[1; 0; 0; 0]
  Mux : Mux  Inputs=2
  Quaternion Multiplication : aerolibutil/Quaternion Multiplication
  Scope : Scope
      settings: ShowLegends=on  SaveName=ScopeData9
  q_o : Outport
  wires:
  omega_o/1 -> Gain/1
  Gain/1 -> Mux/2
  Constant/1 -> Mux/1
  Quaternion Multiplication/1 -> Integrator/1
  Integrator/1 -> Quaternion Multiplication/2, q_o/1, Scope/1
  Mux/1 -> Quaternion Multiplication/1

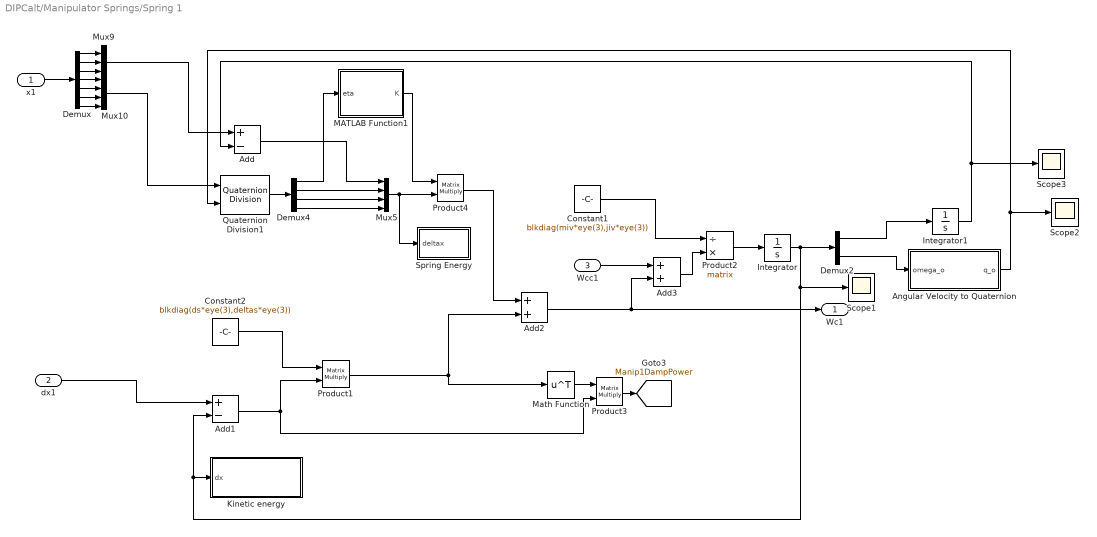
== system DIPCalt/Manipulator Springs/Spring 1 ==
  x1 : Inport
  dx1 : Inport  Port=2
  Wcc1 : Inport  Port=3
  Add : Sum  Inputs=+-
  Add1 : Sum  Inputs=+-
  Add2 : Sum
  Add3 : Sum
  Angular Velocity to Quaternion : Subsystem
  Constant1 : Constant  Value=blkdiag(miv*eye(3),jiv*eye(3))
  Constant2 : Constant  Value=blkdiag(ds*eye(3),deltas*eye(3))
  Demux : Demux  Outputs=7
  Demux2 : Demux  Outputs=2
  Demux4 : Demux
  Integrator : Integrator  InitialCondition=zeros(6,1)
  Integrator1 : Integrator  InitialCondition=r(1:3)
  Kinetic energy : Subsystem
  MATLAB Function1 : MATLAB Function  TreatAsAtomicUnit=on
  Math Function : Math  Operator=transpose  SaturateOnIntegerOverflow=on
  Mux10 : Mux
  Mux5 : Mux
  Mux9 : Mux  Inputs=3
  Product1 : Product  Multiplication=Matrix(*)
  Product2 : Product  Inputs=/*  Multiplication=Matrix(*)
  Product3 : Product  Multiplication=Matrix(*)
  Product4 : Product  Multiplication=Matrix(*)
  Quaternion Division1 : aerolibutil/Quaternion Division
  Scope1 : Scope
      settings: SaveName=ScopeData38
  Scope2 : Scope
      settings: YMin=-0.4  YMax=1  SaveName=ScopeData43
  Scope3 : Scope
      settings: SaveName=ScopeData44
  Spring Energy : Subsystem
  Wc1 : Outport
  tag scope: Manip1DampPower=global
  wires:
  Constant2/1 -> Product1/1
  Add2/1 -> Add3/2, Wc1/1
  x1/1 -> Demux/1
  Demux/1 -> Mux9/1
  Demux/2 -> Mux9/2
  Demux/3 -> Mux9/3
  Demux/4 -> Mux10/1
  Demux/5 -> Mux10/2
  Demux/6 -> Mux10/3
  Demux/7 -> Mux10/4
  MATLAB Function1/1(K) -> Product4/1
  Demux4/1 -> MATLAB Function1/1(eta)
  Add/1 -> Mux5/1
  Demux4/2 -> Mux5/2
  Demux4/3 -> Mux5/3
  Demux4/4 -> Mux5/4
  Quaternion Division1/1 -> Demux4/1
  Mux5/1 -> Spring Energy/1(deltax), Product4/2
  Mux9/1 -> Add/1
  Integrator1/1 -> Scope3/1, Add/2
  Product4/1 -> Add2/1
  Mux10/1 -> Quaternion Division1/1
  Angular Velocity to Quaternion/1(q_o) -> Scope2/1, Quaternion Division1/2
  dx1/1 -> Add1/1
  Add1/1 -> Product1/2, Product3/2
  Constant1/1 -> Product2/1
  Product1/1 -> Add2/2, Math Function/1
  Math Function/1 -> Product3/1
  Product3/1 -> [Manip1DampPower]
  Product2/1 -> Integrator/1
  Add3/1 -> Product2/2
  Integrator/1 -> Demux2/1, Scope1/1, Add1/2, Kinetic energy/1(dx)
  Demux2/2 -> Angular Velocity to Quaternion/1(omega_o)
  Demux2/1 -> Integrator1/1
  Wcc1/1 -> Add3/1

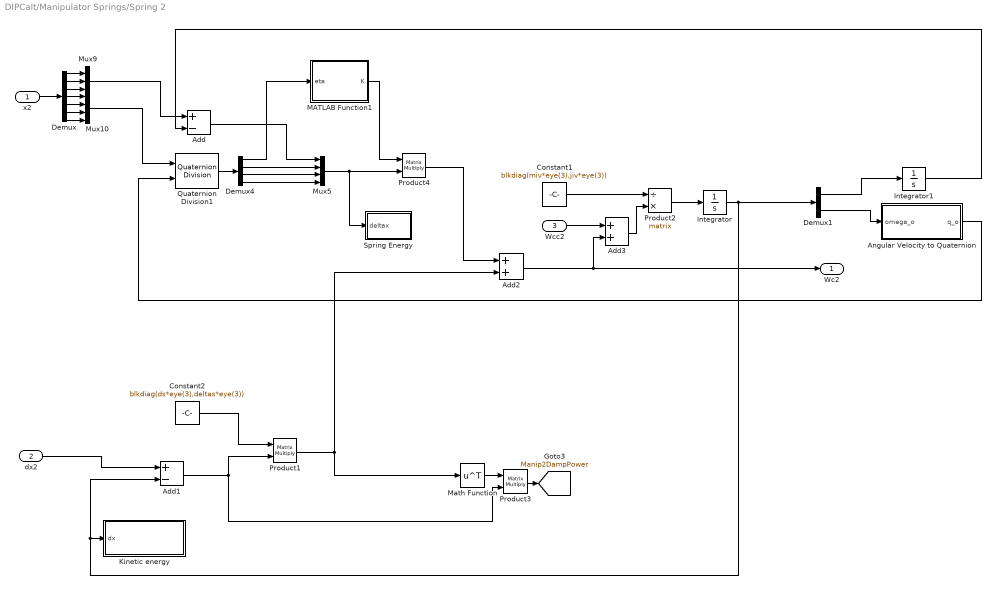
== system DIPCalt/Manipulator Springs/Spring 2 ==
  x2 : Inport
  dx2 : Inport  Port=2
  Wcc2 : Inport  Port=3
  Add : Sum  Inputs=+-
  Add1 : Sum  Inputs=+-
  Add2 : Sum
  Add3 : Sum
  Angular Velocity to Quaternion : Subsystem
  Constant1 : Constant  Value=blkdiag(miv*eye(3),jiv*eye(3))
  Constant2 : Constant  Value=blkdiag(ds*eye(3),deltas*eye(3))
  Demux : Demux  Outputs=7
  Demux1 : Demux  Outputs=2
  Demux4 : Demux
  Integrator : Integrator  InitialCondition=zeros(6,1)
  Integrator1 : Integrator  InitialCondition=r(4:6)
  Kinetic energy : Subsystem
  MATLAB Function1 : MATLAB Function  TreatAsAtomicUnit=on
  Math Function : Math  Operator=transpose  SaturateOnIntegerOverflow=on
  Mux10 : Mux
  Mux5 : Mux
  Mux9 : Mux  Inputs=3
  Product1 : Product  Multiplication=Matrix(*)
  Product2 : Product  Inputs=/*  Multiplication=Matrix(*)
  Product3 : Product  Multiplication=Matrix(*)
  Product4 : Product  Multiplication=Matrix(*)
  Quaternion Division1 : aerolibutil/Quaternion Division
  Spring Energy : Subsystem
  Wc2 : Outport
  tag scope: Manip2DampPower=global
  wires:
  Constant2/1 -> Product1/1
  x2/1 -> Demux/1
  Demux/1 -> Mux9/1
  Demux/2 -> Mux9/2
  Demux/3 -> Mux9/3
  Demux/4 -> Mux10/1
  Demux/5 -> Mux10/2
  Demux/6 -> Mux10/3
  Demux/7 -> Mux10/4
  MATLAB Function1/1(K) -> Product4/1
  Demux4/1 -> MATLAB Function1/1(eta)
  Add/1 -> Mux5/1
  Demux4/2 -> Mux5/2
  Demux4/3 -> Mux5/3
  Demux4/4 -> Mux5/4
  Quaternion Division1/1 -> Demux4/1
  Mux5/1 -> Spring Energy/1(deltax), Product4/2
  Mux9/1 -> Add/1
  Mux10/1 -> Quaternion Division1/1
  Add2/1 -> Add3/2, Wc2/1
  Product4/1 -> Add2/1
  dx2/1 -> Add1/1
  Constant1/1 -> Product2/1
  Add1/1 -> Product1/2, Product3/2
  Product1/1 -> Add2/2, Math Function/1
  Math Function/1 -> Product3/1
  Product3/1 -> [Manip2DampPower]
  Product2/1 -> Integrator/1
  Add3/1 -> Product2/2
  Wcc2/1 -> Add3/1
  Integrator/1 -> Demux1/1, Add1/2, Kinetic energy/1(dx)
  Demux1/2 -> Angular Velocity to Quaternion/1(omega_o)
  Demux1/1 -> Integrator1/1
  Integrator1/1 -> Add/2
  Angular Velocity to Quaternion/1(q_o) -> Quaternion Division1/2

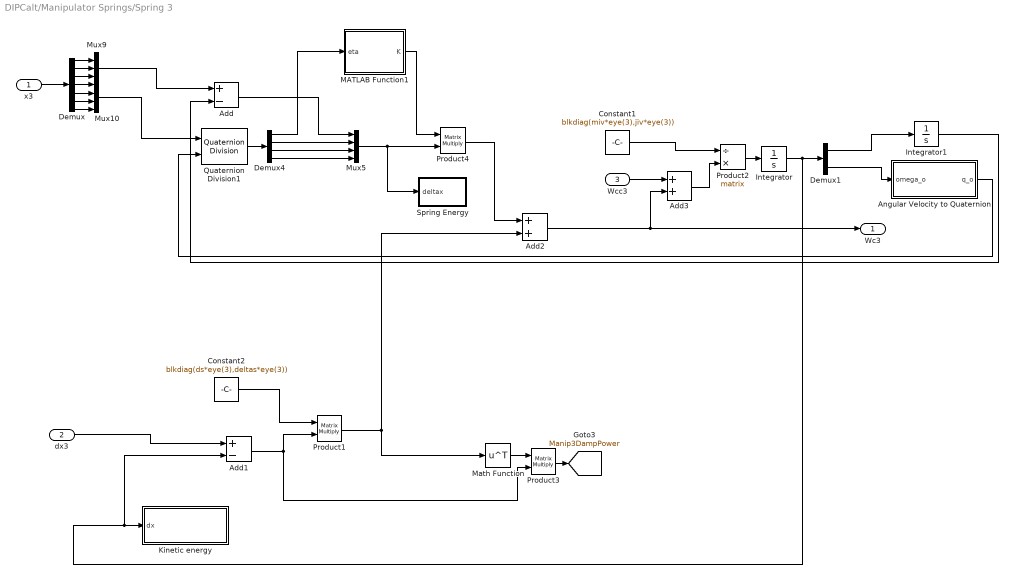
== system DIPCalt/Manipulator Springs/Spring 3 ==
  x3 : Inport
  dx3 : Inport  Port=2
  Wcc3 : Inport  Port=3
  Add : Sum  Inputs=+-
  Add1 : Sum  Inputs=+-
  Add2 : Sum
  Add3 : Sum
  Angular Velocity to Quaternion : Subsystem
  Constant1 : Constant  Value=blkdiag(miv*eye(3),jiv*eye(3))
  Constant2 : Constant  Value=blkdiag(ds*eye(3),deltas*eye(3))
  Demux : Demux  Outputs=7
  Demux1 : Demux  Outputs=2
  Demux4 : Demux
  Integrator : Integrator  InitialCondition=zeros(6,1)
  Integrator1 : Integrator  InitialCondition=r(7:9)
  Kinetic energy : Subsystem
  MATLAB Function1 : MATLAB Function  TreatAsAtomicUnit=on
  Math Function : Math  Operator=transpose  SaturateOnIntegerOverflow=on
  Mux10 : Mux
  Mux5 : Mux
  Mux9 : Mux  Inputs=3
  Product1 : Product  Multiplication=Matrix(*)
  Product2 : Product  Inputs=/*  Multiplication=Matrix(*)
  Product3 : Product  Multiplication=Matrix(*)
  Product4 : Product  Multiplication=Matrix(*)
  Quaternion Division1 : aerolibutil/Quaternion Division
  Spring Energy : Subsystem
  Wc3 : Outport
  tag scope: Manip3DampPower=global
  wires:
  Constant2/1 -> Product1/1
  x3/1 -> Demux/1
  Demux/1 -> Mux9/1
  Demux/2 -> Mux9/2
  Demux/3 -> Mux9/3
  Demux/4 -> Mux10/1
  Demux/5 -> Mux10/2
  Demux/6 -> Mux10/3
  Demux/7 -> Mux10/4
  MATLAB Function1/1(K) -> Product4/1
  Demux4/1 -> MATLAB Function1/1(eta)
  Add/1 -> Mux5/1
  Demux4/2 -> Mux5/2
  Demux4/3 -> Mux5/3
  Demux4/4 -> Mux5/4
  Quaternion Division1/1 -> Demux4/1
  Mux5/1 -> Spring Energy/1(deltax), Product4/2
  Product4/1 -> Add2/1
  Mux9/1 -> Add/1
  Mux10/1 -> Quaternion Division1/1
  dx3/1 -> Add1/1
  Constant1/1 -> Product2/1
  Add1/1 -> Product1/2, Product3/2
  Product1/1 -> Add2/2, Math Function/1
  Math Function/1 -> Product3/1
  Product3/1 -> [Manip3DampPower]
  Product2/1 -> Integrator/1
  Add2/1 -> Add3/2, Wc3/1
  Wcc3/1 -> Add3/1
  Add3/1 -> Product2/2
  Integrator/1 -> Demux1/1, Add1/2, Kinetic energy/1(dx)
  Demux1/2 -> Angular Velocity to Quaternion/1(omega_o)
  Demux1/1 -> Integrator1/1
  Integrator1/1 -> Add/2
  Angular Velocity to Quaternion/1(q_o) -> Quaternion Division1/2

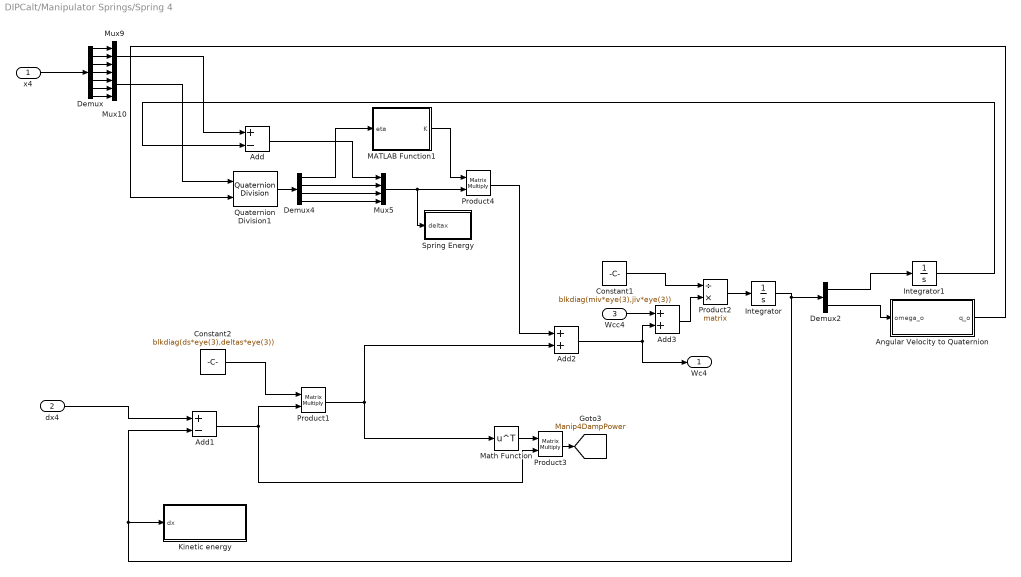
== system DIPCalt/Manipulator Springs/Spring 4 ==
  x4 : Inport
  dx4 : Inport  Port=2
  Wcc4 : Inport  Port=3
  Add : Sum  Inputs=+-
  Add1 : Sum  Inputs=+-
  Add2 : Sum
  Add3 : Sum
  Angular Velocity to Quaternion : Subsystem
  Constant1 : Constant  Value=blkdiag(miv*eye(3),jiv*eye(3))
  Constant2 : Constant  Value=blkdiag(ds*eye(3),deltas*eye(3))
  Demux : Demux  Outputs=7
  Demux2 : Demux  Outputs=2
  Demux4 : Demux
  Integrator : Integrator  InitialCondition=zeros(6,1)
  Integrator1 : Integrator  InitialCondition=r(10:12)
  Kinetic energy : Subsystem
  MATLAB Function1 : MATLAB Function  TreatAsAtomicUnit=on
  Math Function : Math  Operator=transpose  SaturateOnIntegerOverflow=on
  Mux10 : Mux
  Mux5 : Mux
  Mux9 : Mux  Inputs=3
  Product1 : Product  Multiplication=Matrix(*)
  Product2 : Product  Inputs=/*  Multiplication=Matrix(*)
  Product3 : Product  Multiplication=Matrix(*)
  Product4 : Product  Multiplication=Matrix(*)
  Quaternion Division1 : aerolibutil/Quaternion Division
  Spring Energy : Subsystem
  Wc4 : Outport
  tag scope: Manip4DampPower=global
  wires:
  Constant2/1 -> Product1/1
  Add2/1 -> Add3/2, Wc4/1
  x4/1 -> Demux/1
  Demux/1 -> Mux9/1
  Demux/2 -> Mux9/2
  Demux/3 -> Mux9/3
  Demux/4 -> Mux10/1
  Demux/5 -> Mux10/2
  Demux/6 -> Mux10/3
  Demux/7 -> Mux10/4
  Demux4/2 -> Mux5/2
  Demux4/3 -> Mux5/3
  Demux4/4 -> Mux5/4
  Quaternion Division1/1 -> Demux4/1
  Mux5/1 -> Spring Energy/1(deltax), Product4/2
  MATLAB Function1/1(K) -> Product4/1
  Demux4/1 -> MATLAB Function1/1(eta)
  Add/1 -> Mux5/1
  Mux9/1 -> Add/1
  Mux10/1 -> Quaternion Division1/1
  Product4/1 -> Add2/1
  dx4/1 -> Add1/1
  Constant1/1 -> Product2/1
  Add1/1 -> Product1/2, Product3/2
  Product1/1 -> Add2/2, Math Function/1
  Math Function/1 -> Product3/1
  Product3/1 -> [Manip4DampPower]
  Product2/1 -> Integrator/1
  Add3/1 -> Product2/2
  Wcc4/1 -> Add3/1
  Integrator/1 -> Demux2/1, Add1/2, Kinetic energy/1(dx)
  Demux2/2 -> Angular Velocity to Quaternion/1(omega_o)
  Demux2/1 -> Integrator1/1
  Integrator1/1 -> Add/2
  Angular Velocity to Quaternion/1(q_o) -> Quaternion Division1/2

== system DIPCalt/Manipulator motion/Angular Velocity to Quaternion ==
  omega_o : Inport
  Constant : Constant  Value=0
  Gain : Gain  Gain=0.5
  Integrator : Integrator  InitialCondition=[1; 0; 0; 0]
  Mux : Mux  Inputs=2
  Quaternion Multiplication : aerolibutil/Quaternion Multiplication
  Scope : Scope
      settings: ShowLegends=on  SaveName=ScopeData9
  q_o : Outport
  wires:
  omega_o/1 -> Gain/1
  Gain/1 -> Mux/2
  Constant/1 -> Mux/1
  Quaternion Multiplication/1 -> Integrator/1
  Integrator/1 -> Quaternion Multiplication/2, q_o/1, Scope/1
  Mux/1 -> Quaternion Multiplication/1

== system DIPCalt/Object Spring/Angular Velocity to Quaternion ==
  omega_o : Inport
  Constant : Constant  Value=0
  Gain : Gain  Gain=0.5
  Integrator : Integrator  InitialCondition=[1; 0; 0; 0]
  Mux : Mux  Inputs=2
  Quaternion Multiplication : aerolibutil/Quaternion Multiplication
  Scope : Scope
      settings: ShowLegends=on  SaveName=ScopeData9
  q_o : Outport
  wires:
  omega_o/1 -> Gain/1
  Gain/1 -> Mux/2
  Constant/1 -> Mux/1
  Quaternion Multiplication/1 -> Integrator/1
  Integrator/1 -> Quaternion Multiplication/2, q_o/1, Scope/1
  Mux/1 -> Quaternion Multiplication/1

== system DIPCalt/Object Spring/Kinetic energy ==
  dx : Inport
  Constant : Constant  Value=blkdiag(0.5*mv*eye(3),0.5*jv*eye(3))
  Math Function : Math  Operator=transpose  SaturateOnIntegerOverflow=on
  Product : Product  Inputs=3  Multiplication=Matrix(*)
  tag scope: vObjectKineticEnergy=global
  wires:
  dx/1 -> Product/3, Math Function/1
  Math Function/1 -> Product/1
  Constant/1 -> Product/2
  Product/1 -> [vObjectKineticEnergy]

== system DIPCalt/Object Spring/Spring Energy ==
  deltax : Inport
  energy : Inport  Port=2
  Constant : Constant  Commented=on  Value=blkdiag(0.5*kv*eye(3),2*kappav*eye(3))
  MATLAB Function1 : MATLAB Function  TreatAsAtomicUnit=on
  Math Function : Math  Operator=transpose  SaturateOnIntegerOverflow=on
  Product : Product  Inputs=3  Multiplication=Matrix(*)
  tag scope: vObjectSpringEnergy=global
  wires:
  deltax/1 -> Product/3, Math Function/1
  Math Function/1 -> Product/1
  Product/1 -> [vObjectSpringEnergy]
  energy/1 -> MATLAB Function1/1(energy)
  MATLAB Function1/1(K) -> Product/2

== system DIPCalt/Virtual Object Erhart/Angular Velocity to Quaternion ==
  omega_o : Inport
  Constant : Constant  Value=0
  Gain : Gain  Gain=0.5
  Integrator : Integrator  InitialCondition=[1; 0; 0; 0]
  Mux : Mux  Inputs=2
  Quaternion Multiplication : aerolibutil/Quaternion Multiplication
  Scope : Scope
      settings: ShowLegends=on  SaveName=ScopeData9
  q_o : Outport
  wires:
  omega_o/1 -> Gain/1
  Gain/1 -> Mux/2
  Constant/1 -> Mux/1
  Quaternion Multiplication/1 -> Integrator/1
  Integrator/1 -> Quaternion Multiplication/2, q_o/1, Scope/1
  Mux/1 -> Quaternion Multiplication/1

== system DIPCalt/Virtual Object Simulation/Angular Velocity to Quaternion ==
  omega_o : Inport
  Constant : Constant  Value=0
  Gain : Gain  Gain=0.5
  Integrator : Integrator  InitialCondition=[1; 0; 0; 0]
  Mux : Mux  Inputs=2
  Quaternion Multiplication : aerolibutil/Quaternion Multiplication
  Scope : Scope
      settings: ShowLegends=on  SaveName=ScopeData9
  q_o : Outport
  wires:
  omega_o/1 -> Gain/1
  Gain/1 -> Mux/2
  Constant/1 -> Mux/1
  Quaternion Multiplication/1 -> Integrator/1
  Integrator/1 -> Quaternion Multiplication/2, q_o/1, Scope/1
  Mux/1 -> Quaternion Multiplication/1

== system DIPCalt/Virtual Object Simulation1/Angular Velocity to Quaternion ==
  omega_o : Inport
  Constant : Constant  Value=0
  Gain : Gain  Gain=0.5
  Integrator : Integrator  InitialCondition=[1; 0; 0; 0]
  Mux : Mux  Inputs=2
  Quaternion Multiplication : aerolibutil/Quaternion Multiplication
  Scope : Scope
      settings: ShowLegends=on  SaveName=ScopeData9
  q_o : Outport
  wires:
  omega_o/1 -> Gain/1
  Gain/1 -> Mux/2
  Constant/1 -> Mux/1
  Quaternion Multiplication/1 -> Integrator/1
  Integrator/1 -> Quaternion Multiplication/2, q_o/1, Scope/1
  Mux/1 -> Quaternion Multiplication/1

== system DIPCalt/Manipulator Springs/Spring 1/Angular Velocity to Quaternion ==
  omega_o : Inport
  Constant : Constant  Value=0
  Gain : Gain  Gain=0.5
  Integrator : Integrator  InitialCondition=[1; 0; 0; 0]
  Mux : Mux  Inputs=2
  Quaternion Multiplication : aerolibutil/Quaternion Multiplication
  Quaternion Normalize : aerolibutil/Quaternion Normalize
  q_o : Outport
  wires:
  omega_o/1 -> Gain/1
  Gain/1 -> Mux/2
  Constant/1 -> Mux/1
  Quaternion Multiplication/1 -> Integrator/1
  Integrator/1 -> Quaternion Normalize/1
  Mux/1 -> Quaternion Multiplication/1
  Quaternion Normalize/1 -> Quaternion Multiplication/2, q_o/1

== system DIPCalt/Manipulator Springs/Spring 1/Kinetic energy ==
  dx : Inport
  Constant : Constant  Value=blkdiag(0.5*m1*eye(3),0.5*j1*eye(3))
  Math Function : Math  Operator=transpose  SaturateOnIntegerOverflow=on
  Product : Product  Inputs=3  Multiplication=Matrix(*)
  tag scope: Manip1KineticEnergy=global
  wires:
  dx/1 -> Product/3, Math Function/1
  Math Function/1 -> Product/1
  Constant/1 -> Product/2
  Product/1 -> [Manip1KineticEnergy]

== system DIPCalt/Manipulator Springs/Spring 1/Spring Energy ==
  deltax : Inport
  Constant : Constant  Value=blkdiag(0.5*ks*eye(3),2*kappas*eye(3))
  Math Function : Math  Operator=transpose  SaturateOnIntegerOverflow=on
  Product : Product  Inputs=3  Multiplication=Matrix(*)
  tag scope: Manip1SpringEnergy=global
  wires:
  deltax/1 -> Product/3, Math Function/1
  Math Function/1 -> Product/1
  Constant/1 -> Product/2
  Product/1 -> [Manip1SpringEnergy]

== system DIPCalt/Manipulator Springs/Spring 2/Angular Velocity to Quaternion ==
  omega_o : Inport
  Constant : Constant  Value=0
  Gain : Gain  Gain=0.5
  Integrator : Integrator  InitialCondition=[1; 0; 0; 0]
  Mux : Mux  Inputs=2
  Quaternion Multiplication : aerolibutil/Quaternion Multiplication
  Quaternion Normalize : aerolibutil/Quaternion Normalize
  Scope : Scope
      settings: ShowLegends=on  SaveName=ScopeData9
  q_o : Outport
  wires:
  omega_o/1 -> Gain/1
  Gain/1 -> Mux/2
  Constant/1 -> Mux/1
  Quaternion Multiplication/1 -> Integrator/1
  Integrator/1 -> Quaternion Normalize/1
  Mux/1 -> Quaternion Multiplication/1
  Quaternion Normalize/1 -> Quaternion Multiplication/2, q_o/1, Scope/1

== system DIPCalt/Manipulator Springs/Spring 2/Kinetic energy ==
  dx : Inport
  Constant : Constant  Value=blkdiag(0.5*m2*eye(3),0.5*j2*eye(3))
  Math Function : Math  Operator=transpose  SaturateOnIntegerOverflow=on
  Product : Product  Inputs=3  Multiplication=Matrix(*)
  tag scope: Manip2KineticEnergy=global
  wires:
  dx/1 -> Product/3, Math Function/1
  Math Function/1 -> Product/1
  Constant/1 -> Product/2
  Product/1 -> [Manip2KineticEnergy]

== system DIPCalt/Manipulator Springs/Spring 2/Spring Energy ==
  deltax : Inport
  Constant : Constant  Value=blkdiag(0.5*ks*eye(3),2*kappas*eye(3))
  Math Function : Math  Operator=transpose  SaturateOnIntegerOverflow=on
  Product : Product  Inputs=3  Multiplication=Matrix(*)
  tag scope: Manip2SpringEnergy=global
  wires:
  deltax/1 -> Product/3, Math Function/1
  Math Function/1 -> Product/1
  Constant/1 -> Product/2
  Product/1 -> [Manip2SpringEnergy]

== system DIPCalt/Manipulator Springs/Spring 3/Angular Velocity to Quaternion ==
  omega_o : Inport
  Constant : Constant  Value=0
  Gain : Gain  Gain=0.5
  Integrator : Integrator  InitialCondition=[1; 0; 0; 0]
  Mux : Mux  Inputs=2
  Quaternion Multiplication : aerolibutil/Quaternion Multiplication
  Quaternion Normalize : aerolibutil/Quaternion Normalize
  Scope : Scope
      settings: ShowLegends=on  SaveName=ScopeData9
  q_o : Outport
  wires:
  omega_o/1 -> Gain/1
  Gain/1 -> Mux/2
  Constant/1 -> Mux/1
  Quaternion Multiplication/1 -> Integrator/1
  Integrator/1 -> Quaternion Normalize/1
  Mux/1 -> Quaternion Multiplication/1
  Quaternion Normalize/1 -> Quaternion Multiplication/2, q_o/1, Scope/1

== system DIPCalt/Manipulator Springs/Spring 3/Kinetic energy ==
  dx : Inport
  Constant : Constant  Value=blkdiag(0.5*m3*eye(3),0.5*j3*eye(3))
  Math Function : Math  Operator=transpose  SaturateOnIntegerOverflow=on
  Product : Product  Inputs=3  Multiplication=Matrix(*)
  tag scope: Manip3KineticEnergy=global
  wires:
  dx/1 -> Product/3, Math Function/1
  Math Function/1 -> Product/1
  Constant/1 -> Product/2
  Product/1 -> [Manip3KineticEnergy]

== system DIPCalt/Manipulator Springs/Spring 3/Spring Energy ==
  deltax : Inport
  Constant : Constant  Value=blkdiag(0.5*ks*eye(3),2*kappas*eye(3))
  Math Function : Math  Operator=transpose  SaturateOnIntegerOverflow=on
  Product : Product  Inputs=3  Multiplication=Matrix(*)
  tag scope: Manip3SpringEnergy=global
  wires:
  deltax/1 -> Product/3, Math Function/1
  Math Function/1 -> Product/1
  Constant/1 -> Product/2
  Product/1 -> [Manip3SpringEnergy]

== system DIPCalt/Manipulator Springs/Spring 4/Angular Velocity to Quaternion ==
  omega_o : Inport
  Constant : Constant  Value=0
  Gain : Gain  Gain=0.5
  Integrator : Integrator  InitialCondition=[1; 0; 0; 0]
  Mux : Mux  Inputs=2
  Quaternion Multiplication : aerolibutil/Quaternion Multiplication
  Quaternion Normalize : aerolibutil/Quaternion Normalize
  Scope : Scope
      settings: ShowLegends=on  SaveName=ScopeData9
  q_o : Outport
  wires:
  omega_o/1 -> Gain/1
  Gain/1 -> Mux/2
  Constant/1 -> Mux/1
  Quaternion Multiplication/1 -> Integrator/1
  Integrator/1 -> Quaternion Normalize/1
  Mux/1 -> Quaternion Multiplication/1
  Quaternion Normalize/1 -> Quaternion Multiplication/2, q_o/1, Scope/1

== system DIPCalt/Manipulator Springs/Spring 4/Kinetic energy ==
  dx : Inport
  Constant : Constant  Value=blkdiag(0.5*m4*eye(3),0.5*j4*eye(3))
  Math Function : Math  Operator=transpose  SaturateOnIntegerOverflow=on
  Product : Product  Inputs=3  Multiplication=Matrix(*)
  tag scope: Manip4KineticEnergy=global
  wires:
  dx/1 -> Product/3, Math Function/1
  Math Function/1 -> Product/1
  Constant/1 -> Product/2
  Product/1 -> [Manip4KineticEnergy]

== system DIPCalt/Manipulator Springs/Spring 4/Spring Energy ==
  deltax : Inport
  Constant : Constant  Value=blkdiag(0.5*ks*eye(3),2*kappas*eye(3))
  Math Function : Math  Operator=transpose  SaturateOnIntegerOverflow=on
  Product : Product  Inputs=3  Multiplication=Matrix(*)
  tag scope: Manip4SpringEnergy=global
  wires:
  deltax/1 -> Product/3, Math Function/1
  Math Function/1 -> Product/1
  Constant/1 -> Product/2
  Product/1 -> [Manip4SpringEnergy]

== matlab function DIPCalt/Virtual Object Simulation/Centripetal Force ==
  data: dx input; b output; rv parameter; x input
function b = centripetalforce(dx,rv,x)
b = [skew_sm(dx(4:6))*skew_sm(dx(4:6))*quatrot(x(4:7),rv(1:3));
     zeros(3,1);
     skew_sm(dx(4:6))*skew_sm(dx(4:6))*quatrot(x(4:7),rv(4:6));
     zeros(3,1);
     skew_sm(dx(4:6))*skew_sm(dx(4:6))*quatrot(x(4:7),rv(7:9));
     zeros(3,1);
     skew_sm(dx(4:6))*skew_sm(dx(4:6))*quatrot(x(4:7),rv(10:12));
     zeros(3,1)];

== matlab function DIPCalt/Interaction dynamics1/MATLAB Function ==
  data: r parameter; A output; x input
function A = ConstraintMatrix(r,x)
A = [-eye(3) skew_sm(quatrot(x(4:7),r(1:3))) eye(3) zeros(3,21);
        zeros(3) -eye(3) zeros(3) eye(3) zeros(3,18);
        -eye(3) skew_sm(quatrot(x(4:7),r(4:6))) zeros(3,6) eye(3) zeros(3,15);
        zeros(3) -eye(3) zeros(3,9) eye(3) zeros(3,12);
        -eye(3) skew_sm(quatrot(x(4:7),r(7:9))) zeros(3,12) eye(3) zeros(3,9);
        zeros(3) -eye(3) zeros(3,15) eye(3) zeros(3,6);
        -eye(3) skew_sm(quatrot(x(4:7),r(10:12))) zeros(3,18) eye(3) zeros(3);
        zeros(3) -eye(3) zeros(3,21) eye(3)];

== matlab function DIPCalt/Interaction dynamics1/Centripetal Force ==
  data: dx input; b output; r parameter; x input
function b = centripetalforce(dx,r,x)
b = [skew_sm(dx(4:6))*skew_sm(dx(4:6))*quatrot(x(4:7),r(1:3));
     zeros(3,1);
     skew_sm(dx(4:6))*skew_sm(dx(4:6))*quatrot(x(4:7),r(4:6));
     zeros(3,1);
     skew_sm(dx(4:6))*skew_sm(dx(4:6))*quatrot(x(4:7),r(7:9));
     zeros(3,1);
     skew_sm(dx(4:6))*skew_sm(dx(4:6))*quatrot(x(4:7),r(10:12));
     zeros(3,1)];

== matlab function DIPCalt/Interaction dynamics1/Coriolis Force ==
  data: dx input; hcoriolis output; j0 parameter; m0 parameter
function hcoriolis = CoriolisForce(dx,j0,m0)
hcoriolis = [m0*skew_sm(dx(4:6))*dx(1:3);
        j0*skew_sm(dx(4:6))*dx(4:6)];

== matlab function DIPCalt/Manipulator Springs/Spring 1/MATLAB Function1 ==
  data: eta input; K output; ks parameter; kappas parameter
function K = stiffness(eta,ks,kappas)
K = blkdiag(ks*eye(3),2*eta*kappas*eye(3));

== matlab function DIPCalt/Manipulator Springs/Spring 2/MATLAB Function1 ==
  data: eta input; K output; ks parameter; kappas parameter
function K = stiffness(eta,ks,kappas)
K = blkdiag(ks*eye(3),2*eta*kappas*eye(3));

== matlab function DIPCalt/Manipulator Springs/Spring 3/MATLAB Function1 ==
  data: eta input; K output; ks parameter; kappas parameter
function K = stiffness(eta,ks,kappas)
K = blkdiag(ks*eye(3),2*eta*kappas*eye(3));

== matlab function DIPCalt/Manipulator Springs/Spring 4/MATLAB Function1 ==
  data: eta input; K output; ks parameter; kappas parameter
function K = stiffness(eta,ks,kappas)
K = blkdiag(ks*eye(3),2*eta*kappas*eye(3));
